simulink model "twoDoF_I_PDandFF"  (R2019b)
settings: Solver=VariableStepAuto  StartTime=0.0  StopTime=10.0  RelTol=1e-3
undefined symbols (not defined in the file): Kd, Kff, Ki, Kp, w, z
settings Model: Creator=Student  LastModifiedBy=Student

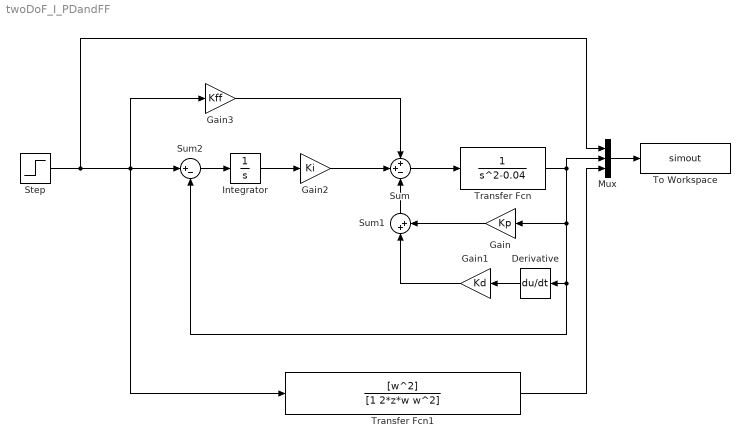
== system twoDoF_I_PDandFF ==
  Derivative : Derivative
  Gain : Gain  Gain=Kp
  Gain1 : Gain  Gain=Kd
  Gain2 : Gain  Gain=Ki
  Gain3 : Gain  Gain=Kff
  Integrator : Integrator
  Mux : Mux  Inputs=3
  Step : Step  Time=0  SampleTime=0
  Sum : Sum  Inputs=++-
  Sum1 : Sum  Inputs=|++
  Sum2 : Sum  Inputs=|+-
  To Workspace : ToWorkspace  VariableName=simout  SaveFormat=Timeseries  SampleTime=-1
  Transfer Fcn : TransferFcn  Denominator=[1 0 -0.04]
  Transfer Fcn1 : TransferFcn  Numerator=[w^2]  Denominator=[1 2*z*w w^2]
  wires:
  Transfer Fcn/1 -> Sum2/2, Derivative/1, Gain/1, Mux/2
  Step/1 -> Gain3/1, Sum2/1, Transfer Fcn1/1, Mux/1
  Mux/1 -> To Workspace/1
  Derivative/1 -> Gain1/1
  Gain/1 -> Sum1/2
  Gain1/1 -> Sum1/1
  Sum/1 -> Transfer Fcn/1
  Integrator/1 -> Gain2/1
  Sum2/1 -> Integrator/1
  Transfer Fcn1/1 -> Mux/3
  Gain2/1 -> Sum/2
  Sum1/1 -> Sum/3
  Gain3/1 -> Sum/1
